simulink model "ControlVelocidad_Observador_MotorDC"  (R2020b)
settings: Solver=VariableStepAuto  StartTime=0.0  StopTime=10  RelTol=1e-3
libraries: fl_lib x6, nesl_utility x4, ee_lib x1, pid_lib x1
settings Model: Creator=petir  LastModifiedBy=petir
settings SolverCC: AlgebraicLoopSolver=LineSearch

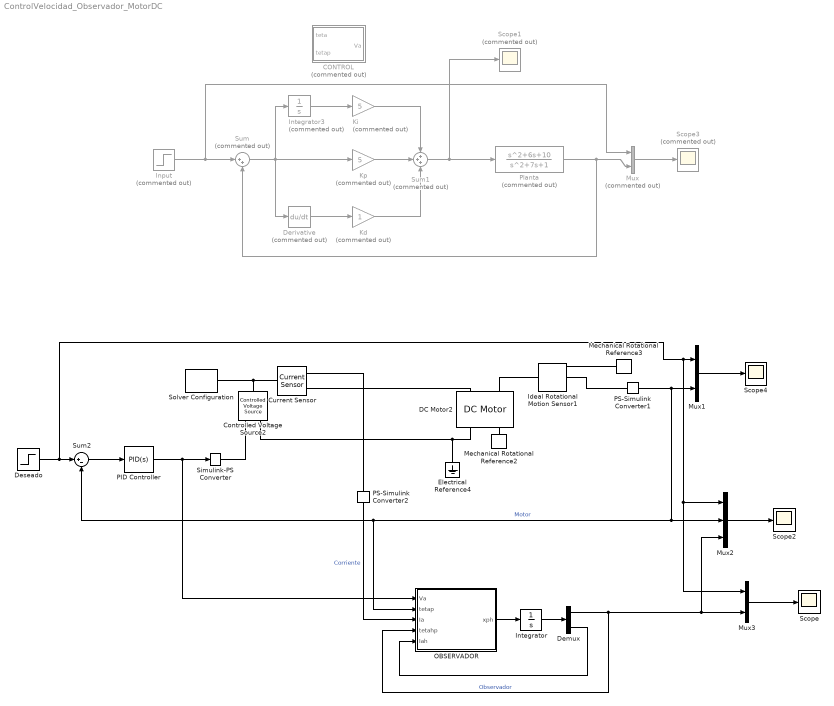
== system ControlVelocidad_Observador_MotorDC ==
  CONTROL : MATLAB Function  Commented=on  TreatAsAtomicUnit=on
  Controlled Voltage Source2 : fl_lib/Electrical/Electrical Sources/Controlled Voltage Source
  Current Sensor : fl_lib/Electrical/Electrical Sensors/Current Sensor
  DC Motor2 : ee_lib/Electromechanical/Brushed Motors/DC Motor  field_option=ee.enum.field_option.pm  Rf=100 Ohm  Lf=1 H  Laf=0.15 H  If0=0 A  parameterization=ee.enum.dcparam_option.circuit_param  Ra=8.3 Ohm  La=1.51e-3 H  emf_or_torque=ee.enum.emf_or_torque.ki  Kv=0.0879 V/(rad/s)  Ki=0.0879 N*m/A  T_stall=0.24e-3 N*m  w_max=19100 rpm  w_rated=15000 rpm  P_rated=0.08 W  V_rated=1.5 V  J=80.7e-6 kg*m^2  lam_param=ee.enum.lam_param.damping  lam=14.41e-6 N*m/(rad/s)  i_noload=0 A  V_i_noload=1.5 V  speed0=0 rpm  enable_fault_armature=ee.enum.faults.faultEnable.no  rev_faulted=1 / 3  G_faulted_armature=1e-5 S  fault_trigger_armature=ee.enum.faults.faultTrigger.temporal  t_fault_armature=1 s  max_permissible_current_armature=inf A  t_fail_on_current_armature=1 s  enable_fault_field=ee.enum.faults.faultEnable.no  G_faulted_field=1e-5 S  fault_trigger_field=ee.enum.faults.faultTrigger.temporal  t_fault_field=1 s  max_permissible_current_field=inf A  t_fail_on_current_field=1 s  fault_action=ee.enum.faults.faultAction.none  alpha=3.93e-3 1/K  Tmeas=25 degC  thermal_mass=100 J/K  initial_temperature=25 degC
  Demux : Demux  Outputs=2
  Derivative : Derivative  Commented=on
  Deseado : Step  After=pi/2  SampleTime=0
  Electrical Reference4 : fl_lib/Electrical/Electrical Elements/Electrical Reference
  Ideal Rotational Motion Sensor1 : fl_lib/Mechanical/Mechanical Sensors/Ideal Rotational Motion Sensor  wrap_angle=simscape.enum.onoff.off  offset=0 rad
  Input : Step  Commented=on  SampleTime=0
  Integrator : Integrator
  Integrator3 : Integrator  Commented=on
  Kd : Gain  Commented=on
  Ki : Gain  Commented=on  Gain=5
  Kp : Gain  Commented=on  Gain=5
  Mechanical Rotational Reference2 : fl_lib/Mechanical/Rotational Elements/Mechanical Rotational Reference
  Mechanical Rotational Reference3 : fl_lib/Mechanical/Rotational Elements/Mechanical Rotational Reference
  Mux : Mux  Commented=on  Inputs=2
  Mux1 : Mux  Inputs=2
  Mux2 : Mux  Inputs=3
  Mux3 : Mux  Inputs=2
  OBSERVADOR : MATLAB Function  TreatAsAtomicUnit=on
  PID Controller : pid_lib/PID Controller  Controller=PID  Form=Ideal  TimeDomain=Continuous-time  UseExternalTs=off  SampleTime=-1  IntegratorMethod=Forward Euler  FilterMethod=Forward Euler  ControllerParametersSource=internal  P=5  I=3  D=1  UseFilter=on  N=100  TunerSelectOption=Transfer Function Based (PID Tuner App)  InitialConditionSource=internal  InitialConditionForIntegrator=0  InitialConditionForFilter=0  DifferentiatorICPrevScaledInput=0  ExternalReset=none  TrackingMode=off  Kt=1  LimitOutput=off  SatLimitsSource=internal  UpperSaturationLimit=inf  LowerSaturationLimit=-inf  LinearizeAsGain=on  AntiWindupMode=none  Kb=1  POutMin=[]  POutMax=[]  IOutMin=[]  IOutMax=[]  DOutMin=[]  DOutMax=[]  NOutMin=[]  NOutMax=[]  SumOutMin=[]  SumOutMax=[]  SaturationOutMin=[]  SaturationOutMax=[]  PParamMin=[]  PParamMax=[]  IParamMin=[]  IParamMax=[]  DParamMin=[]  DParamMax=[]  NParamMin=[]  NParamMax=[]  KbParamMin=[]  KbParamMax=[]  KtParamMin=[]  KtParamMax=[]  KbOutMin=[]  KbOutMax=[]  KtOutMin=[]  KtOutMax=[]  IntegratorOutMin=[]  IntegratorOutMax=[]  FilterOutMin=[]  FilterOutMax=[]  SumI1OutMin=[]  SumI1OutMax=[]  SumI2OutMin=[]  SumI2OutMax=[]  SumI3OutMin=[]  SumI3OutMax=[]  SumI4OutMin=[]  SumI4OutMax=[]  SumDOutMin=[]  SumDOutMax=[]  DifferentiatorOutMin=[]  DifferentiatorOutMax=[]  FilterDiffOutCoefMin=[]  FilterDiffOutCoefMax=[]  ReciprocalOutMin=[]  ReciprocalOutMax=[]  SumDenOutMin=[]  SumDenOutMax=[]  SumNumOutMin=[]  SumNumOutMax=[]  DivideOutMin=[]  DivideOutMax=[]  UdiffTsProdOutMin=[]  UdiffTsProdOutMax=[]  NTsProdOutMin=[]  NTsProdOutMax=[]  UintegralTsProdOutMin=[]  UintegralTsProdOutMax=[]  UngainTsProdOutMin=[]  UngainTsProdOutMax=[]  IntegratorContinuousStateAttributes=''  IntegratorStateMustResolveToSignalObject=off  IntegratorRTWStateStorageClass=Auto  FilterContinuousStateAttributes=''  FilterStateMustResolveToSignalObject=off  FilterRTWStateStorageClass=Auto  ParallelPVariant=Passthrough  IdealPVariant=InternalParameters  IVariant=InternalParameters  DVariant=InternalParameters  IntegratorVariant=Continuous  SatVariant=Disabled  AWVariant=Passthrough  PCopyVariant=Disabled  TRVariant=Disabled  FdbkBlocksVariant=Forward  IdealPFdbkVariant=Disabled  SatFdbkVariant=Disabled  DerivativeFilterVariant=ContFilter  NVariant=InternalParameters  NCopyVariant=Disabled  FilterICVariant=InternalICsFilter  IntegratorICVariant=InternalICs  ExternalResetVariant=Disabled  TRSumVariant=Passthrough  SumFdbkVariant=Disabled  SumVariant=Sum_PID  TsampFilterVariant=InternalTs  TsampNgainVariant=Passthrough  TsampIntegralVariant=Passthrough  ExternalSaturationOutDataTypeStr=Inherit: Same as second input
  PS-Simulink Converter1 : nesl_utility/PS-Simulink Converter  PhysicalDomain=network_engine_domain  SubClassName=ps_output  LeftPortType=input  RightPortType=output  PseudoPeriodic=off  Frequencies=[]  Unit=inherit  AffineConversion=off
  PS-Simulink Converter2 : nesl_utility/PS-Simulink Converter  PhysicalDomain=network_engine_domain  SubClassName=ps_output  LeftPortType=input  RightPortType=output  PseudoPeriodic=off  Frequencies=[]  Unit=inherit  AffineConversion=off
  Planta : TransferFcn  Commented=on  Numerator=[1 6 10]  Denominator=[1 7 1]
  Scope : Scope
  Scope1 : Scope  Commented=on
  Scope2 : Scope
  Scope3 : Scope  Commented=on
  Scope4 : Scope
  Simulink-PS Converter : nesl_utility/Simulink-PS Converter  PhysicalDomain=network_engine_domain  SubClassName=ps_input  LeftPortType=input  RightPortType=output  PseudoPeriodic=off  Frequencies=[]  NoiseDistribution=none  NoiseParameters=[]  Unit=1  AffineConversion=off  FilteringAndDerivatives=provide  SimscapeFilterOrder=1  InputFilterTimeConstant=0.001  UdotUserProvided=0
  Solver Configuration : nesl_utility/Solver Configuration  PhysicalDomain=network_engine_domain  SubClassName=solver  LeftPortType=input  RightPortType=generic  Tones=[]  Harmonics=[]  SimulateNoise=off  Profile=off  UseLocalSampling=off  EnableSwitchedLinearOptims=on  FrequencyDomain=off  UseCCode=off  RelTol=0.001  AbsTol=1e-06  MinStep=1e-09  ToWorkspace=off  RevertToSquareIcSolve=off  NumHomotopyIterations=100  PhasorMode=off  PhasorModeNumHarmonics=1  DoDC=off  ResidualTolerance=1e-09  UseLocalSolver=off  LocalSolverChoice=NE_BACKWARD_EULER_ADVANCER  LocalSolverSampleTime=0.001  DoFixedCost=off  MaxNonlinIter=3  MaxModeIter=2  ComputeImpulses=off  ImpulseIterations=2  LinearAlgebra=auto  EquationFormulation=NE_TIME_EF  DelaysMemoryBudget=1024  AutomaticFiltering=on  FilteringTimeConstant=0.001  PartitionStorageMethod=AS_NEEDED  PartitionMemoryBudget=1024  PartitionMethod=ROBUST
  Sum : Sum  Commented=on  Inputs=|++
  Sum1 : Sum  Commented=on  Inputs=+++
  Sum2 : Sum  Inputs=|+-
  wires:
  Input/1 -> Mux/1, Sum/1
  Sum/1 -> Derivative/1, Integrator3/1, Kp/1
  Sum1/1 -> Planta/1, Scope1/1
  Kp/1 -> Sum1/2
  Integrator3/1 -> Ki/1
  Ki/1 -> Sum1/1
  Derivative/1 -> Kd/1
  Kd/1 -> Sum1/3
  OBSERVADOR/1(xph) -> Integrator/1
  Planta/1 -> Mux/2, Sum/2
  Mux/1 -> Scope3/1
  Mux1/1 -> Scope4/1
  PID Controller/1 -> OBSERVADOR/1(Va), Simulink-PS Converter/1
  Sum2/1 -> PID Controller/1
  PS-Simulink Converter1/1 -> Mux1/2, OBSERVADOR/2(tetap), Sum2/2, Mux2/2  "Motor"
  Deseado/1 -> Mux3/1, Mux2/1, Mux1/1, Sum2/1
  Mux2/1 -> Scope2/1
  PS-Simulink Converter2/1 -> OBSERVADOR/3(Ia)  "Corriente"
  Integrator/1 -> Demux/1
  Demux/2 -> OBSERVADOR/5(Iah)
  Demux/1 -> Mux2/3, Mux3/2, OBSERVADOR/4(tetahp)  "Observador"
  Mux3/1 -> Scope/1
  connections:
  Controlled Voltage Source2/RConn2 -- DC Motor2/RConn1 -- Electrical Reference4/LConn1
  Solver Configuration/RConn1 -- Current Sensor/LConn1 -- Controlled Voltage Source2/LConn1
  DC Motor2/LConn2 -- Ideal Rotational Motion Sensor1/LConn1
  Ideal Rotational Motion Sensor1/RConn1 -- Mechanical Rotational Reference3/LConn1
  PS-Simulink Converter1/LConn1 -- Ideal Rotational Motion Sensor1/RConn2
  DC Motor2/RConn2 -- Mechanical Rotational Reference2/LConn1
  Simulink-PS Converter/RConn1 -- Controlled Voltage Source2/RConn1
  Current Sensor/RConn2 -- DC Motor2/LConn1
  PS-Simulink Converter2/LConn1 -- Current Sensor/RConn1

== matlab function ControlVelocidad_Observador_MotorDC/CONTROL ==
  data: teta input; Va output; tetap input
function Va = fcn(teta, tetap)
% Parametros
Ra = 8.3;
Ke = 0.0879;
Ki = 0.0879;
J = 80.7e-6;
B = 14.41e-6;
TL = 0.1;

tetad = 2 * pi;
Kp = 5;
Kd = 2;

Vaux = Kp * (tetad - teta) - Kd * tetap;
Va = J * Ra / Ki * (Vaux + Ki * Ke / (J * Ra) * tetap + B / J * tetap + 1 / J * TL);

== matlab function ControlVelocidad_Observador_MotorDC/OBSERVADOR ==
  data: Va input; xph output; tetap input; Ia input; tetahp input; Iah input
function xph = fcn(Va, tetap, Ia, tetahp, Iah)
% Parámetros
Ra = 8.3;
La = 1.51e-3;
Ke = 0.0879;
Ki = 0.0879;
J = 80.7e-6;
B = 14.41e-6;

A = [-B / J, Ki / J; -Ke/La, -Ra / La];
B_mat = [0; 1 / La];
C = [0, 1];

x = [tetap; Ia];
xh = [tetahp; Iah];

y = C * x;
yh = C * xh;

K = [19.8214; 96.8214];

% xph = Axh + Bu + k(y-yh)
xph = A * xh + B_mat * Va + K * (y - yh);
